simulink model "Non_Linear_Plant_LQR"  (R2024b)
settings: Solver=VariableStepAuto  StartTime=0.0  StopTime=300  RelTol=1e-3
settings Model: Creator=aryaman  LastModifiedBy=aryaman
settings DataIOCC: SaveFormat=StructureWithTime

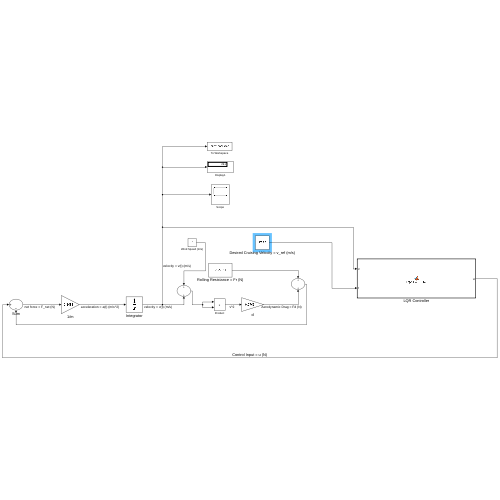
[thumbnail: Simulink's stored preview of the top-level diagram]
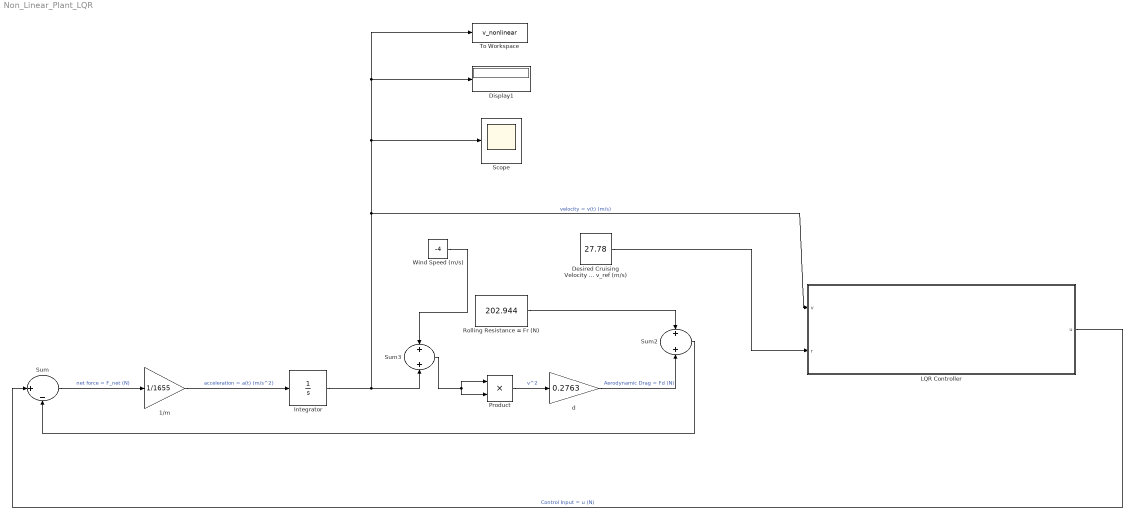
== system Non_Linear_Plant_LQR ==
  1/m : Gain  Gain=1/1655
  Desired Cruising Velocity = v_ref (m/s) : Constant  Value=27.78
  Display1 : Display
  Integrator : Integrator
  LQR Controller : MATLAB Function  TreatAsAtomicUnit=on
  Product : Product
  Rolling Resistance = Fr (N) : Constant  Value=202.944
  Scope : Scope
  Sum : Sum  Inputs=||+|-
  Sum2 : Sum  Inputs=+|+
  Sum3 : Sum  Inputs=+|+
  To Workspace : ToWorkspace  VariableName=v_nonlinear  SampleTime=-1
  Wind Speed (m/s) : Constant  Value=-4
  d : Gain  Gain=0.2763
  wires:
  Sum/1 -> 1/m/1  "net force = F_net (N)"
  1/m/1 -> Integrator/1  "acceleration = a(t) (m/s^2)"
  Integrator/1 -> Sum3/2, LQR Controller/1(v), Scope/1, Display1/1, To Workspace/1  "velocity = v(t) (m/s)"
  Desired Cruising Velocity = v_ref (m/s)/1 -> LQR Controller/2(r)
  LQR Controller/1(u) -> Sum/1  "Control Input = u (N)"
  Product/1 -> d/1  "v^2"
  Rolling Resistance = Fr (N)/1 -> Sum2/1
  d/1 -> Sum2/2  "Aerodynamic Drag = Fd (N)"
  Sum2/1 -> Sum/2
  Wind Speed (m/s)/1 -> Sum3/1
  Sum3/1 -> Product/1, Product/2

== matlab function Non_Linear_Plant_LQR/LQR Controller ==
  data: v input; u output; r input
function u = LQR_Controller(v, r)
K = 33.9944;
Nbar = 49.3555;

u = -K * v + Nbar * r;
end
